simulink model "quantiser1bit"  (Simulink 8.1)
settings: Solver=FixedStepDiscrete  StartTime=0.0  StopTime=250  RelTol=1e-3
libraries: dspsrcs4 x2
settings Model: Creator=amyles  LastModifiedBy=amyles
settings DataIOCC: MaxDataPoints=50000
settings DebuggingCC: StrictBusMsg=Warning

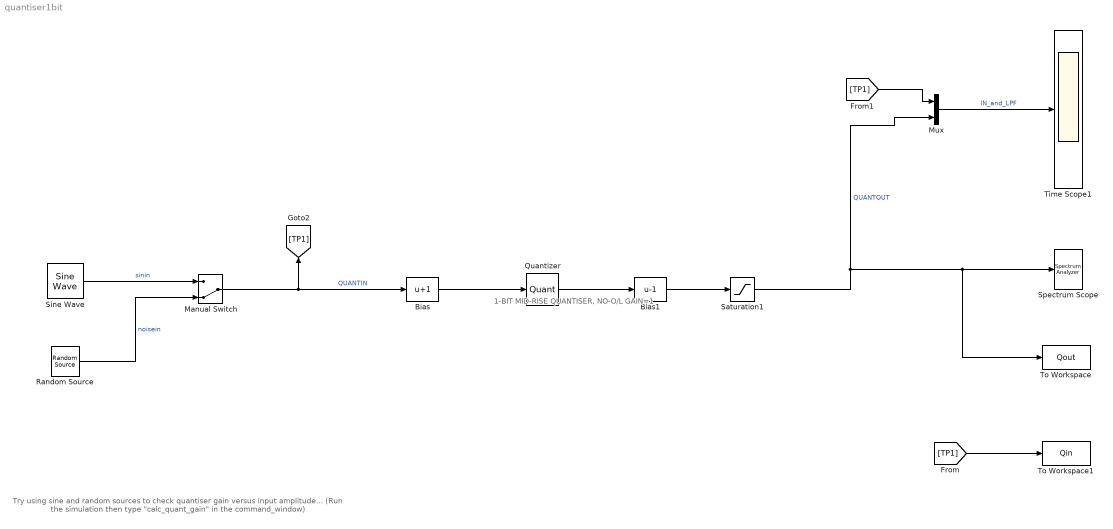
== system quantiser1bit ==
  note: 1-BIT MID-RISE QUANTISER, NO-O/L GAIN=1
  note: Try using sine and random
      | sources to check quantiser
      | gain versus input amplitude...
      |
      | (Run the simulation then
      | type "calc_quant_gain" in the
      | command_window)
  Bias : Bias  Bias=1
      settings: AttributesFormatString=Need offset to give\nMID-RISE quantiser
  Bias1 : Bias  Bias=-1
      settings: AttributesFormatString=Shift outputs to\n...,-3,-1,1,3,...
  Manual Switch : ManualSwitch  CurrentSetting=0
  Mux : Mux  Inputs=2
  Quantizer : Quantizer  QuantizationInterval=2  LinearizeAsGain=off
      settings: AttributesFormatString=Interval set to 2, so get\noutputs ..., -4, -2, 0, 2, 4,...
  Random Source : dspsrcs4/Random Source  SrcType=Uniform  NormMethod=Ziggurat  CltLength=12  MinVal=-1.5  MaxVal=1.5  MeanVal=0  VarVal=1  RepMode=Not repeatable  rawSeed=1  IsInherit=off  SampMode=Discrete  SampTime=1/100  SampFrame=1  DataType=Double  OutComplex=Real
  Saturation1 : Saturate  UpperLimit=1  LowerLimit=-1
      settings: AttributesFormatString=Limit quantiser\noutput to +/-1
  Sine Wave : dspsrcs4/Sine Wave  Amplitude=1.05  Frequency=0.005  Phase=0  SampleMode=Discrete  OutComplex=Real  CompMethod=Trigonometric fcn  TableSize=Speed  SampleTime=1/100  SamplesPerFrame=1  ResetState=Restart at time zero  dataType=double  wordLen=16  udDataType=sfix(16)  fracBitsMode=Best precision  numFracBits=15  OutDataTypeStr=double  LastOutDataTypeStr=double
  Spectrum Scope : SpectrumAnalyzer
      settings: CopyFcn=scopeextensions.ScopeBlock.callback(gcbh, 'onBlockCopy', gcbh);  DeleteFcn=scopeextensions.ScopeBlock.callback(gcbh, 'onBlockDelete');  PreSaveFcn=scopeextensions.ScopeBlock.callback(gcbh, 'onModelSave');  NameChangeFcn=scopeextensions.ScopeBlock.callback(gcbh, 'onBlockRename');  CloseFcn=scopeextensions.ScopeBlock.callback(gcbh, 'onBlockClose');  PreDeleteFcn=scopeextensions.ScopeBlock.callback(gcbh, 'onBlockPreDelete');
  Time Scope1 : Scope
      settings: TimeRange=250  DataFormat=Structure  MaxDataPoints=100000
  To Workspace : ToWorkspace  VariableName=Qout  SampleTime=-1
      settings: AttributesFormatString=Export SDM output\nto workspace for\npost-processing
  To Workspace1 : ToWorkspace  VariableName=Qin  SampleTime=-1
      settings: AttributesFormatString=Export Quant' input\nto workspace for\npost-processing\n(e.g quantiser gain)
  wires:
  Bias/1 -> Quantizer/1
  Saturation1/1 -> To Workspace/1, Spectrum Scope/1, Mux/2  "QUANTOUT"
  Quantizer/1 -> Bias1/1
  Bias1/1 -> Saturation1/1
  Mux/1 -> Time Scope1/1  "IN_and_LPF"
  [TP1] -> To Workspace1/1
  [TP1] -> Mux/1
  Manual Switch/1 -> Bias/1, [TP1]  "QUANTIN"
  Sine Wave/1 -> Manual Switch/1  "sinin"
  Random Source/1 -> Manual Switch/2  "noisein"
